simulink model "noxiebo"  (R2018b)
settings: Solver=FixedStepDiscrete  StartTime=0.0  StopTime=Inf  FixedStep=Auto  RelTol=1e-3  EnableMultiTasking=on
model workspace (MAT data in the model file):
  encoderResolution = 4096
  indexOffset = 0
  polePairs = 16
undefined symbols (not defined in the file or in its folder): Down, Up
libraries: idelinklib_common x37, c2833xlib x7, c280xlib x6, simulink x3, simulink_extras x2, c2000lib x1
(part 2 of 3)

== system noxiebo/Subsystem1/PI-Nr ==
  err : Inport
  reset : Inport  Port=2
  P : Inport  Port=3
  I : Inport  Port=4
  D : Inport  Port=5
  OV : Inport  Port=6
  Constant1 : Constant  Value=0  OutDataTypeStr=Inherit: Inherit via back propagation
  Constant2 : Constant  Value=25  OutDataTypeStr=Inherit: Inherit via back propagation
  Constant3 : Constant  Value=0  OutDataTypeStr=Inherit: Inherit via back propagation
  Constant5 : Constant  Value=0  OutDataTypeStr=Inherit: Inherit via back propagation
  Logical Operator5 : Logic  AllPortsSameDT=off  OutDataTypeStr=boolean
  Logical Operator6 : Logic  Operator=NOT  AllPortsSameDT=off  OutDataTypeStr=boolean
  Product : Product  RndMeth=Zero
  Product1 : Product  RndMeth=Zero
  Product2 : Product  RndMeth=Zero
  RC filter8 : Subsystem  mask{a=0.4}
      mask prompts: a "Time Constant"
  Saturation : Saturate  UpperLimit=max  LowerLimit=min  LinearizeAsGain=off  ZeroCross=off  OutDataTypeStr=double
  Saturation1 : Saturate  UpperLimit=ermax  LowerLimit=ermin  LinearizeAsGain=off  ZeroCross=off  OutDataTypeStr=double
  Saturation2 : Saturate  UpperLimit=max  LowerLimit=min  LinearizeAsGain=off  ZeroCross=off  OutDataTypeStr=double
  Sum1 : Sum  Inputs=+++
  Sum2 : Sum  Inputs=+-
  Sum4 : Sum
  Switch{1..4} (4 alike) : Switch  Criteria=u2 > Threshold  SaturateOnIntegerOverflow=on  InputSameDT=on
  Unit Delay1 : UnitDelay  SampleTime=-1
  Unit Delay3 : UnitDelay  SampleTime=-1
  out : Outport
  wires:
  Logical Operator6/1 -> Logical Operator5/2
  Logical Operator5/1 -> Switch4/2
  RC filter8/1(y) -> Sum1/3
  Constant3/1 -> Switch3/3
  Switch3/1 -> Switch1/3
  Saturation2/1 -> Switch3/1
  Switch1/1 -> out/1
  OV/1 -> Logical Operator6/1, Switch1/2
  Constant2/1 -> Switch1/1
  Sum1/1 -> Saturation2/1
  Product2/1 -> RC filter8/1(x)
  Unit Delay1/1 -> Sum2/2
  D/1 -> Product2/2
  Sum2/1 -> Product2/1
  Switch4/1 -> Unit Delay3/1
  Unit Delay3/1 -> Sum4/2
  Saturation/1 -> Switch4/1, Sum1/2
  Sum4/1 -> Saturation/1
  Product1/1 -> Sum4/1
  I/1 -> Product1/2
  Product/1 -> Sum1/1
  Saturation1/1 -> Switch2/1
  err/1 -> Saturation1/1
  Constant1/1 -> Switch2/3
  reset/1 -> Logical Operator5/1, Switch3/2, Switch2/2
  Switch2/1 -> Unit Delay1/1, Sum2/1, Product1/1, Product/1
  P/1 -> Product/2
  Constant5/1 -> Switch4/3

== system noxiebo/Subsystem1/RC filter1 ==
  x : Inport
  Constant2 : Constant  Value=a  OutDataTypeStr=double
  Constant3 : Constant  Value=1-a  OutDataTypeStr=double
  Divide : Product
  Divide1 : Product
  Sum2 : Sum
  Unit Delay2 : UnitDelay  SampleTime=-1
  y : Outport
  wires:
  x/1 -> Divide/1
  Constant2/1 -> Divide/2
  Constant3/1 -> Divide1/1
  Divide/1 -> Sum2/1
  Divide1/1 -> Sum2/2
  Sum2/1 -> y/1, Unit Delay2/1
  Unit Delay2/1 -> Divide1/2

== system noxiebo/Subsystem1/RC filter2 ==
  x : Inport
  Constant2 : Constant  Value=a  OutDataTypeStr=double
  Constant3 : Constant  Value=1-a  OutDataTypeStr=double
  Divide : Product
  Divide1 : Product
  Sum2 : Sum
  Unit Delay2 : UnitDelay  SampleTime=-1
  y : Outport
  wires:
  Unit Delay2/1 -> Divide1/2
  Sum2/1 -> Unit Delay2/1, y/1
  Divide1/1 -> Sum2/2
  Divide/1 -> Sum2/1
  Constant3/1 -> Divide1/1
  Constant2/1 -> Divide/2
  x/1 -> Divide/1

== system noxiebo/Subsystem1/RC filter3 ==
  x : Inport
  Constant2 : Constant  Value=a  OutDataTypeStr=double
  Constant3 : Constant  Value=1-a  OutDataTypeStr=double
  Divide : Product
  Divide1 : Product
  Sum2 : Sum
  Unit Delay2 : UnitDelay  SampleTime=-1
  y : Outport
  wires:
  Unit Delay2/1 -> Divide1/2
  Sum2/1 -> Unit Delay2/1, y/1
  Divide1/1 -> Sum2/2
  Divide/1 -> Sum2/1
  Constant3/1 -> Divide1/1
  Constant2/1 -> Divide/2
  x/1 -> Divide/1

== system noxiebo/Subsystem1/RC filter4 ==
  x : Inport
  Constant2 : Constant  Value=a  OutDataTypeStr=double
  Constant3 : Constant  Value=1-a  OutDataTypeStr=double
  Divide : Product
  Divide1 : Product
  Sum2 : Sum
  Unit Delay2 : UnitDelay  SampleTime=-1
  y : Outport
  wires:
  x/1 -> Divide/1
  Constant2/1 -> Divide/2
  Constant3/1 -> Divide1/1
  Divide/1 -> Sum2/1
  Divide1/1 -> Sum2/2
  Sum2/1 -> y/1, Unit Delay2/1
  Unit Delay2/1 -> Divide1/2

== system noxiebo/Subsystem1/RC filter5 ==
  x : Inport
  Constant2 : Constant  Value=a  OutDataTypeStr=double
  Constant3 : Constant  Value=1-a  OutDataTypeStr=double
  Divide : Product
  Divide1 : Product
  Sum2 : Sum
  Unit Delay2 : UnitDelay  SampleTime=-1
  y : Outport
  wires:
  Unit Delay2/1 -> Divide1/2
  Sum2/1 -> Unit Delay2/1, y/1
  Divide1/1 -> Sum2/2
  Divide/1 -> Sum2/1
  Constant3/1 -> Divide1/1
  Constant2/1 -> Divide/2
  x/1 -> Divide/1

== system noxiebo/Subsystem1/RC filter9 ==
  x : Inport
  Constant2 : Constant  Value=a  OutDataTypeStr=double
  Constant3 : Constant  Value=1-a  OutDataTypeStr=double
  Divide : Product
  Divide1 : Product
  Sum2 : Sum
  Unit Delay2 : UnitDelay  SampleTime=-1
  y : Outport
  wires:
  Unit Delay2/1 -> Divide1/2
  Sum2/1 -> Unit Delay2/1, y/1
  Divide1/1 -> Sum2/2
  Divide/1 -> Sum2/1
  Constant3/1 -> Divide1/1
  Constant2/1 -> Divide/2
  x/1 -> Divide/1

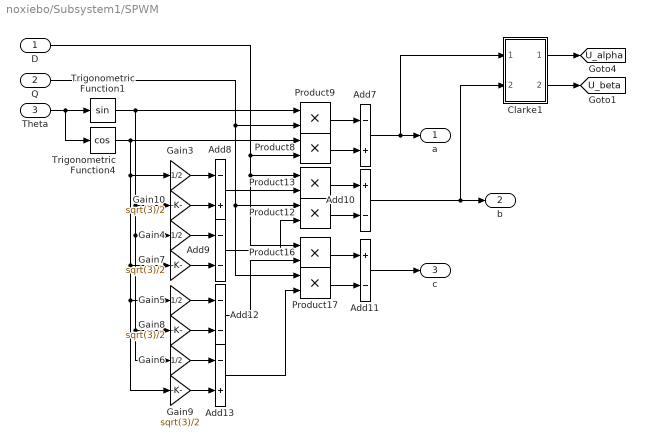
== system noxiebo/Subsystem1/SPWM ==
  D : Inport
  Q : Inport  Port=2
  Theta : Inport  Port=3
  Add10 : Sum  Inputs=+-
  Add11 : Sum  Inputs=+-
  Add12 : Sum  Inputs=--
  Add13 : Sum  Inputs=-+
  Add7 : Sum  Inputs=-+
  Add8 : Sum  Inputs=-+
  Add9 : Sum  Inputs=--
  Clarke1 : Subsystem
  Gain{7..10} (4 alike) : Gain  Gain=sqrt(3)/2
  Gain{3..6} (4 alike) : Gain  Gain=1/2
  Product{8..9,12..13,16..17} (6 alike) : Product  RndMeth=Zero
  Trigonometric Function1 : Trigonometry
  Trigonometric Function4 : Trigonometry  Operator=cos
  a : Outport
  b : Outport  Port=2
  c : Outport  Port=3
  tag scope: U_alpha=global, U_beta=global
  wires:
  Theta/1 -> Trigonometric Function1/1, Trigonometric Function4/1
  Trigonometric Function4/1 -> Product8/1, Gain3/1, Gain5/1, Gain9/1, Gain7/1
  Product8/1 -> Add7/2
  Trigonometric Function1/1 -> Product9/1, Gain4/1, Gain6/1, Gain8/1, Gain10/1
  Product9/1 -> Add7/1
  Gain3/1 -> Add8/1
  Gain4/1 -> Add9/1
  Gain7/1 -> Add9/2
  Product13/1 -> Add10/1
  Product12/1 -> Add10/2
  Add8/1 -> Product13/2
  Add9/1 -> Product12/2
  Product16/1 -> Add11/1
  Product17/1 -> Add11/2
  Add12/1 -> Product16/2
  Add13/1 -> Product17/2
  Add7/1 -> a/1, Clarke1/1(In1)
  Add10/1 -> b/1, Clarke1/2(In2)
  Add11/1 -> c/1
  Gain6/1 -> Add13/1
  Gain8/1 -> Add12/2
  Gain5/1 -> Add12/1
  Gain9/1 -> Add13/2
  Gain10/1 -> Add8/2
  D/1 -> Product8/2, Product13/1, Product16/1
  Q/1 -> Product9/2, Product12/1, Product17/1
  Clarke1/1(alpha) -> [U_alpha]
  Clarke1/2(beta) -> [U_beta]

== system noxiebo/Subsystem1/SPWM_5 ==
  D : Inport
  Q : Inport  Port=2
  Theta : Inport  Port=3
  Add10 : Sum  Inputs=+-
  Add11 : Sum  Inputs=+-
  Add12 : Sum  Inputs=--
  Add13 : Sum  Inputs=-+
  Add7 : Sum  Inputs=-+
  Add8 : Sum  Inputs=-+
  Add9 : Sum  Inputs=--
  Gain{7..10} (4 alike) : Gain  Gain=sqrt(3)/2
  Gain{3..6} (4 alike) : Gain  Gain=1/2
  Product{8..9,12..13,16..17} (6 alike) : Product  RndMeth=Zero
  Trigonometric Function1 : Trigonometry
  Trigonometric Function4 : Trigonometry  Operator=cos
  a : Outport
  b : Outport  Port=2
  c : Outport  Port=3
  wires:
  Q/1 -> Product17/1, Product12/1, Product9/2
  D/1 -> Product16/1, Product13/1, Product8/2
  Gain10/1 -> Add8/2
  Gain9/1 -> Add13/2
  Gain5/1 -> Add12/1
  Gain8/1 -> Add12/2
  Gain6/1 -> Add13/1
  Add11/1 -> c/1
  Add10/1 -> b/1
  Add7/1 -> a/1
  Add13/1 -> Product17/2
  Add12/1 -> Product16/2
  Product17/1 -> Add11/2
  Product16/1 -> Add11/1
  Add9/1 -> Product12/2
  Add8/1 -> Product13/2
  Product12/1 -> Add10/2
  Product13/1 -> Add10/1
  Gain7/1 -> Add9/2
  Gain4/1 -> Add9/1
  Gain3/1 -> Add8/1
  Product9/1 -> Add7/1
  Trigonometric Function1/1 -> Gain10/1, Gain8/1, Gain6/1, Gain4/1, Product9/1
  Product8/1 -> Add7/2
  Trigonometric Function4/1 -> Gain7/1, Gain9/1, Gain5/1, Gain3/1, Product8/1
  Theta/1 -> Trigonometric Function4/1, Trigonometric Function1/1

== system noxiebo/Subsystem1/SPWM_7 ==
  D : Inport
  Q : Inport  Port=2
  Theta : Inport  Port=3
  Add10 : Sum  Inputs=+-
  Add11 : Sum  Inputs=+-
  Add12 : Sum  Inputs=--
  Add13 : Sum  Inputs=-+
  Add7 : Sum  Inputs=-+
  Add8 : Sum  Inputs=-+
  Add9 : Sum  Inputs=--
  Gain{7..10} (4 alike) : Gain  Gain=sqrt(3)/2
  Gain{3..6} (4 alike) : Gain  Gain=1/2
  Product{8..9,12..13,16..17} (6 alike) : Product  RndMeth=Zero
  Trigonometric Function1 : Trigonometry
  Trigonometric Function4 : Trigonometry  Operator=cos
  a : Outport
  b : Outport  Port=2
  c : Outport  Port=3
  wires:
  Q/1 -> Product17/1, Product12/1, Product9/2
  D/1 -> Product16/1, Product13/1, Product8/2
  Gain10/1 -> Add8/2
  Gain9/1 -> Add13/2
  Gain5/1 -> Add12/1
  Gain8/1 -> Add12/2
  Gain6/1 -> Add13/1
  Add11/1 -> c/1
  Add10/1 -> b/1
  Add7/1 -> a/1
  Add13/1 -> Product17/2
  Add12/1 -> Product16/2
  Product17/1 -> Add11/2
  Product16/1 -> Add11/1
  Add9/1 -> Product12/2
  Add8/1 -> Product13/2
  Product12/1 -> Add10/2
  Product13/1 -> Add10/1
  Gain7/1 -> Add9/2
  Gain4/1 -> Add9/1
  Gain3/1 -> Add8/1
  Product9/1 -> Add7/1
  Trigonometric Function1/1 -> Gain10/1, Gain8/1, Gain6/1, Gain4/1, Product9/1
  Product8/1 -> Add7/2
  Trigonometric Function4/1 -> Gain7/1, Gain9/1, Gain5/1, Gain3/1, Product8/1
  Theta/1 -> Trigonometric Function4/1, Trigonometric Function1/1

== system noxiebo/Subsystem1/Subsystem2 ==
  In1 : Inport
  In2 : Inport  Port=2
  Product : Product  RndMeth=Zero
  Product1 : Product  RndMeth=Zero
  Sqrt : Sqrt  SaturateOnIntegerOverflow=on
  Sum17 : Sum
  Out1 : Outport
  wires:
  Product/1 -> Sum17/1
  Product1/1 -> Sum17/2
  Sum17/1 -> Sqrt/1
  In1/1 -> Product/2, Product/1
  In2/1 -> Product1/2, Product1/1
  Sqrt/1 -> Out1/1

== system noxiebo/Subsystem1/abc//dq current ==
  iga : Inport
  igb : Inport  Port=2
  angle : Inport  Port=3
  Clarke1 : Subsystem
  Park1 : Subsystem
  igd : Outport
  igq : Outport  Port=2
  tag scope: i_alpha=global, i_beta=global
  wires:
  Park1/1(d) -> igd/1
  iga/1 -> Clarke1/1(In1)
  Park1/2(q) -> igq/1
  igb/1 -> Clarke1/2(In2)
  Clarke1/1(alpha) -> Park1/1(alpha), [i_alpha]
  Clarke1/2(beta) -> Park1/2(beta), [i_beta]
  angle/1 -> Park1/3(theta)

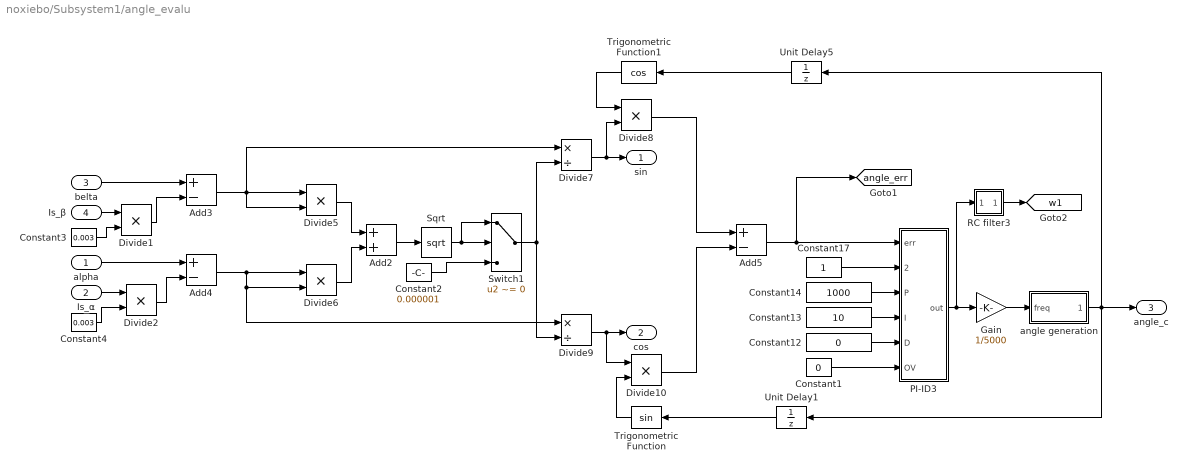
== system noxiebo/Subsystem1/angle_evalu ==
  alpha : Inport
  Is_α : Inport  Port=2
  belta : Inport  Port=3
  Is_β : Inport  Port=4
  Add2 : Sum
  Add3 : Sum  Inputs=+-
  Add4 : Sum  Inputs=+-
  Add5 : Sum  Inputs=+-
  Constant1 : Constant  Value=0  OutDataTypeStr=double
  Constant12 : Constant  Value=0  OutDataTypeStr=double
  Constant13 : Constant  Value=10  OutDataTypeStr=double
  Constant14 : Constant  Value=1000  OutDataTypeStr=double
  Constant17 : Constant  OutDataTypeStr=double
  Constant2 : Constant  Value=0.000001  OutDataTypeStr=double
  Constant3 : Constant  Value=0.003  OutDataTypeStr=double
  Constant4 : Constant  Value=0.003  OutDataTypeStr=double
  Divide{1..2,5..6,8,10} (6 alike) : Product  Inputs=**
  Divide7 : Product  Inputs=*/
  Divide9 : Product  Inputs=*/
  Gain : Gain  Gain=1/5000
  PI-ID3 : Subsystem  mask{ermax=0.5*pi, ermin=-0.5*pi, max=500, min=-500}
      mask prompts: ermax "Err max limit"; ermin "Err min limit"; max "Output max limit"; min "Output min limit"
  RC filter3 : Subsystem  mask{a=0.8}
      mask prompts: a "Time Constant"
  Sqrt : Sqrt  SaturateOnIntegerOverflow=on
  Switch1 : Switch  Criteria=u2 ~= 0
  Trigonometric Function : Trigonometry
  Trigonometric Function1 : Trigonometry  Operator=cos
  Unit Delay1 : UnitDelay  SampleTime=-1
  Unit Delay5 : UnitDelay  SampleTime=-1
  angle generation : Subsystem
  sin : Outport
  cos : Outport  Port=2
  angle_c : Outport  Port=3
  tag scope: angle_err=global, w1=global
  wires:
  belta/1 -> Add3/1
  Add3/1 -> Divide5/1, Divide5/2, Divide7/1
  Divide1/1 -> Add3/2
  Divide2/1 -> Add4/2
  Is_β/1 -> Divide1/1
  Is_α/1 -> Divide2/1
  Add4/1 -> Divide6/1, Divide6/2, Divide9/1
  Divide5/1 -> Add2/1
  Divide6/1 -> Add2/2
  Add2/1 -> Sqrt/1
  Divide7/1 -> sin/1, Divide8/2
  Divide9/1 -> cos/1, Divide10/1
  Trigonometric Function/1 -> Divide10/2
  Divide8/1 -> Add5/1
  Divide10/1 -> Add5/2
  Add5/1 -> PI-ID3/1(err), [angle_err]
  Constant17/1 -> PI-ID3/2(reset)
  Constant12/1 -> PI-ID3/5(D)
  Constant1/1 -> PI-ID3/6(OV)
  Constant14/1 -> PI-ID3/3(P)
  Constant13/1 -> PI-ID3/4(I)
  Gain/1 -> angle generation/1(freq)
  PI-ID3/1(out) -> Gain/1, RC filter3/1(x)
  angle generation/1(angle_0) -> Unit Delay5/1, Unit Delay1/1, angle_c/1
  Unit Delay5/1 -> Trigonometric Function1/1
  Unit Delay1/1 -> Trigonometric Function/1
  Trigonometric Function1/1 -> Divide8/1
  Sqrt/1 -> Switch1/2, Switch1/1
  Constant2/1 -> Switch1/3
  Switch1/1 -> Divide7/2, Divide9/2
  RC filter3/1(y) -> [w1]
  alpha/1 -> Add4/1
  Constant3/1 -> Divide1/2
  Constant4/1 -> Divide2/2

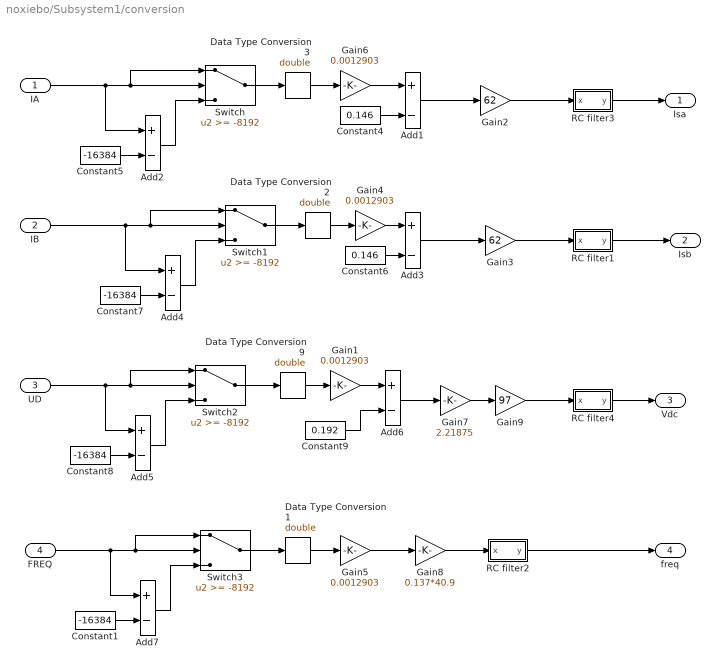
== system noxiebo/Subsystem1/conversion ==
  IA : Inport
  IB : Inport  Port=2
  UD : Inport  Port=3
  FREQ : Inport  Port=4
  Add{1..7} (7 alike) : Sum  Inputs=+-
  Constant{1,5,7..8} (4 alike) : Constant  Value=-16384  OutDataTypeStr=int16
  Constant4 : Constant  Value=0.146  OutDataTypeStr=double
  Constant6 : Constant  Value=0.146  OutDataTypeStr=double
  Constant9 : Constant  Value=0.192  OutDataTypeStr=double
  Data Type Conversion{1..3,9} (4 alike) : DataTypeConversion  OutDataTypeStr=double
  Gain{1,4..6} (4 alike) : Gain  Gain=0.0012903
  Gain2 : Gain  Gain=62
  Gain3 : Gain  Gain=62
  Gain7 : Gain  Gain=2.21875
  Gain8 : Gain  Gain=0.137*40.9
  Gain9 : Gain  Gain=97
  RC filter1 : Subsystem  mask{a=0.2}
      mask prompts: a "Time Constant"
  RC filter2 : Subsystem  mask{a=0.1}
      mask prompts: a "Time Constant"
  RC filter3 : Subsystem  mask{a=0.2}
      mask prompts: a "Time Constant"
  RC filter4 : Subsystem  mask{a=0.1}
      mask prompts: a "Time Constant"
  Switch{,1..3} (4 alike) : Switch  Threshold=-8192
  Isa : Outport
  Isb : Outport  Port=2
  Vdc : Outport  Port=3
  freq : Outport  Port=4
  wires:
  UD/1 -> Switch2/1, Switch2/2, Add5/1
  IA/1 -> Switch/1, Switch/2, Add2/1
  Constant5/1 -> Add2/2
  Add2/1 -> Switch/3
  Switch/1 -> Data Type Conversion3/1
  Data Type Conversion3/1 -> Gain6/1
  Gain2/1 -> RC filter3/1(x)
  Add1/1 -> Gain2/1
  Gain6/1 -> Add1/1
  Constant4/1 -> Add1/2
  IB/1 -> Switch1/1, Switch1/2, Add4/1
  Constant7/1 -> Add4/2
  Add4/1 -> Switch1/3
  Switch1/1 -> Data Type Conversion2/1
  Data Type Conversion2/1 -> Gain4/1
  Add3/1 -> Gain3/1
  Gain4/1 -> Add3/1
  Constant6/1 -> Add3/2
  Data Type Conversion9/1 -> Gain1/1
  Gain7/1 -> Gain9/1
  Constant8/1 -> Add5/2
  Add5/1 -> Switch2/3
  Switch2/1 -> Data Type Conversion9/1
  Gain1/1 -> Add6/1
  Add6/1 -> Gain7/1
  Constant9/1 -> Add6/2
  FREQ/1 -> Switch3/1, Switch3/2, Add7/1
  Data Type Conversion1/1 -> Gain5/1
  Constant1/1 -> Add7/2
  Add7/1 -> Switch3/3
  Switch3/1 -> Data Type Conversion1/1
  Gain5/1 -> Gain8/1
  RC filter2/1(y) -> freq/1
  Gain8/1 -> RC filter2/1(x)
  RC filter1/1(y) -> Isb/1
  RC filter3/1(y) -> Isa/1
  RC filter4/1(y) -> Vdc/1
  Gain9/1 -> RC filter4/1(x)
  Gain3/1 -> RC filter1/1(x)

== system noxiebo/Subsystem1/dq_5 ==
  alpha : Inport
  beta : Inport  Port=2
  theta : Inport  Port=3
  Add4 : Sum
  Add5 : Sum
  Gain1 : Gain  Gain=-1
  Product{,1..3} (4 alike) : Product  RndMeth=Zero
  cos : Trigonometry  Operator=cos
  sin : Trigonometry
  d : Outport
  q : Outport  Port=2
  wires:
  sin/1 -> Product2/1, Product/1
  beta/1 -> Product3/2, Product/2
  cos/1 -> Product3/1, Product1/2
  Add5/1 -> q/1
  theta/1 -> sin/1, cos/1
  Add4/1 -> d/1
  alpha/1 -> Product2/2, Product1/1
  Product1/1 -> Add4/1
  Product/1 -> Add4/2
  Product2/1 -> Gain1/1
  Gain1/1 -> Add5/1
  Product3/1 -> Add5/2

== system noxiebo/Subsystem1/dq_7 ==
  alpha : Inport
  beta : Inport  Port=2
  theta : Inport  Port=3
  Add4 : Sum
  Add5 : Sum
  Gain1 : Gain  Gain=-1
  Product{,1..3} (4 alike) : Product  RndMeth=Zero
  cos : Trigonometry  Operator=cos
  sin : Trigonometry
  d : Outport
  q : Outport  Port=2
  wires:
  sin/1 -> Product2/1, Product/1
  beta/1 -> Product3/2, Product/2
  cos/1 -> Product3/1, Product1/2
  Add5/1 -> q/1
  theta/1 -> sin/1, cos/1
  Add4/1 -> d/1
  alpha/1 -> Product2/2, Product1/1
  Product1/1 -> Add4/1
  Product/1 -> Add4/2
  Product2/1 -> Gain1/1
  Gain1/1 -> Add5/1
  Product3/1 -> Add5/2

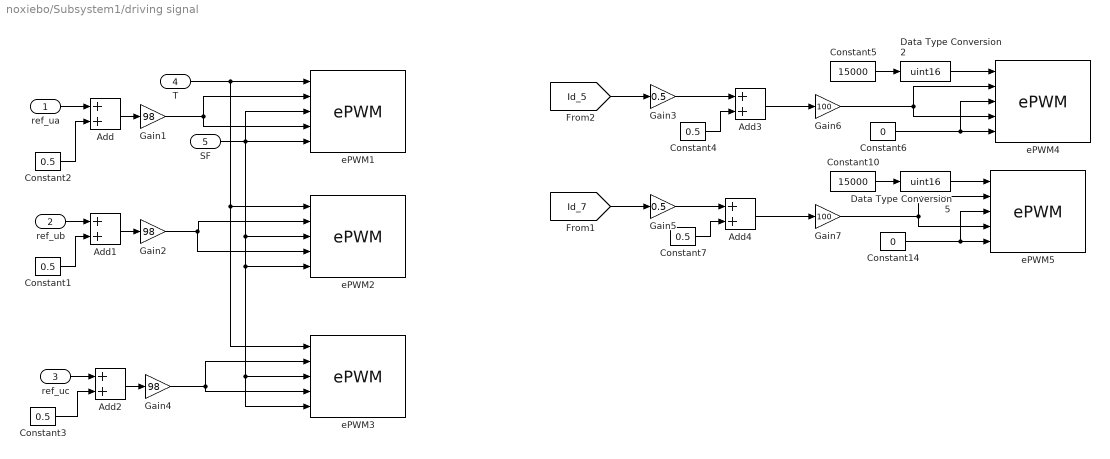
== system noxiebo/Subsystem1/driving signal ==
  ref_ua : Inport
  ref_ub : Inport  Port=2
  ref_uc : Inport  Port=3
  T : Inport  Port=4
  SF : Inport  Port=5
  Add{,1..4} (5 alike) : Sum
  Constant{1..4,7} (5 alike) : Constant  Value=0.5  OutDataTypeStr=double
  Constant10 : Constant  Value=15000  OutDataTypeStr=int16
  Constant14 : Constant  Value=0  OutDataTypeStr=boolean
  Constant5 : Constant  Value=15000  OutDataTypeStr=int16
  Constant6 : Constant  Value=0  OutDataTypeStr=boolean
  Data Type Conversion2 : DataTypeConversion  OutDataTypeStr=uint16
  Data Type Conversion5 : DataTypeConversion  OutDataTypeStr=uint16
  Gain1 : Gain  Gain=98
  Gain2 : Gain  Gain=98
  Gain3 : Gain  Gain=0.5
  Gain4 : Gain  Gain=98
  Gain5 : Gain  Gain=0.5
  Gain6 : Gain  Gain=100
  Gain7 : Gain  Gain=100
  ePWM1 : c280xlib/ePWM  checkMode=off  useModule=ePWM1  periodUnits=Clock cycles  timerSource=Input port  timerPeriod_clk=15000  timerPeriod_sec=1/20000  tbshadow=Counter equals to zero  countingMode=Up-Down  phaseActiveEnable=Disable  phaseDirection=Count down after sync  phaseActive=0  synchronizationEnable=off  synchronizationOption=Counter equals to zero (CTR=Zero)  clockPrescale=1  HSclockPrescale=1  ePWMxAStatus=off  CMPAUnits=Percentages  CMPASource=Input port  CMPAValue_per=0  CMPAValue_clk=32000  enCMPAshadow=Counter equals to zero  ePWMxAactionLogic1=Do nothing  ePWMxAactionLogic2=Do nothing  ePWMxAactionLogic3=Clear  ePWMxAactionLogic4=Set  ePWMxAactionLogic5=Do nothing  ePWMxAactionLogic6=Do nothing  ePWMxALoadMode=Load on counter equals to zero (CTR=Zero)  ePWMxACSFenable=on  ePWMxACSFvalue=Forcing disable  ePWMxASFreload=Zero  enHRPWM=off  HRPWM_LoadMode=Counter equals to zero (CTR=ZERO)  HRPWM_CTLMode=Phase control mode  HRPWM_EDGMode=Both edge  enSFO=on  ePWMxBStatus=on  CMPBUnits=Percentages  CMPBSource=Input port  CMPBValue_per=0  CMPBValue_clk=32000  enCMPBshadow=Counter equals to zero  ePWMxBactionLogic1=Do nothing  ePWMxBactionLogic2=Do nothing  ePWMxBactionLogic3=Do nothing  ePWMxBactionLogic4=Do nothing  ePWMxBactionLogic5=Set  ePWMxBactionLogic6=Clear  ePWMxBLoadMode=Load on counter equals to zero (CTR=Zero)  ePWMxBCSFenable=on  ePWMxBCSFvalue=Forcing disable  ePWMxBSFreload=Zero  enableDBePWMxA=on  enableDBePWMxB=on  DBpolarity=Active high complementary (AHC)  DBedgeDelay=Positive  DBSource_ePWMxA=ePWMxB  DBSource_ePWMxB=ePWMxB  DBperiodSource=Specify via dialog  REDperiod=525  FEDperiod=525  adcstartModuleA=off  adcrequestEventA=First event  adcstartEventA=Counter equals to zero (CTR=Zero)  adcstartModuleB=off  adcrequestEventB=First event  adcstartEventB=Counter equals to zero (CTR=Zero)  intEn=on  intPrd=First event  intSel=Counter equals to zero (CTR=Zero)  chopperEnable=off  chopperFrequency=1  chopperFirstwidth=1  chopperDuty=12.5%  tripZonesource=Specify via dialog  tzselOSHT1=off  tzselOSHT2=off  tzselOSHT3=off  tzselOSHT4=off  tzselOSHT5=off  tzselOSHT6=off  tzselCBC1=off  tzselCBC2=off  tzselCBC3=off  tzselCBC4=off  tzselCBC5=off  tzselCBC6=off  enTzOstIntr=off  enTzCbcIntr=off  ePWMxAforced=No action  ePWMxBforced=No action  timerPeriod=-1  ePWMxAValue=0  ePWMxBValue=0  tripZoneoption=One-shot trip (OSHT)
      settings: SourceProductName=Embedded Coder Support Package for Texas Instruments C2000 Processors  SourceProductBaseCode=TIC2000
  ePWM2 : c280xlib/ePWM  checkMode=off  useModule=ePWM2  periodUnits=Clock cycles  timerSource=Input port  timerPeriod_clk=15000  timerPeriod_sec=1/20000  tbshadow=Counter equals to zero  countingMode=Up-Down  phaseActiveEnable=Set counter to phase value specified via dialog  phaseDirection=Count up after sync  phaseActive=0  synchronizationEnable=off  synchronizationOption=Pass through (EPWMxSYNCI or SWFSYNC)  clockPrescale=1  HSclockPrescale=1  ePWMxAStatus=off  CMPAUnits=Percentages  CMPASource=Input port  CMPAValue_per=0  CMPAValue_clk=32000  enCMPAshadow=Counter equals to zero  ePWMxAactionLogic1=Do nothing  ePWMxAactionLogic2=Do nothing  ePWMxAactionLogic3=Clear  ePWMxAactionLogic4=Set  ePWMxAactionLogic5=Do nothing  ePWMxAactionLogic6=Do nothing  ePWMxALoadMode=Load on counter equals to zero (CTR=Zero)  ePWMxACSFenable=on  ePWMxACSFvalue=Forcing disable  ePWMxASFreload=Zero  enHRPWM=off  HRPWM_LoadMode=Counter equals to zero (CTR=ZERO)  HRPWM_CTLMode=Phase control mode  HRPWM_EDGMode=Both edge  enSFO=on  ePWMxBStatus=on  CMPBUnits=Percentages  CMPBSource=Input port  CMPBValue_per=0  CMPBValue_clk=32000  enCMPBshadow=Counter equals to zero  ePWMxBactionLogic1=Do nothing  ePWMxBactionLogic2=Do nothing  ePWMxBactionLogic3=Do nothing  ePWMxBactionLogic4=Do nothing  ePWMxBactionLogic5=Set  ePWMxBactionLogic6=Clear  ePWMxBLoadMode=Load on counter equals to zero (CTR=Zero)  ePWMxBCSFenable=on  ePWMxBCSFvalue=Forcing disable  ePWMxBSFreload=Zero  enableDBePWMxA=on  enableDBePWMxB=on  DBpolarity=Active high complementary (AHC)  DBedgeDelay=Positive  DBSource_ePWMxA=ePWMxB  DBSource_ePWMxB=ePWMxB  DBperiodSource=Specify via dialog  REDperiod=525  FEDperiod=525  adcstartModuleA=off  adcrequestEventA=First event  adcstartEventA=Counter equals to zero (CTR=Zero)  adcstartModuleB=off  adcrequestEventB=First event  adcstartEventB=Counter equals to zero (CTR=Zero)  intEn=off  intPrd=First event  intSel=Counter equals to zero (CTR=Zero)  chopperEnable=off  chopperFrequency=1  chopperFirstwidth=1  chopperDuty=12.5%  tripZonesource=Specify via dialog  tzselOSHT1=off  tzselOSHT2=off  tzselOSHT3=off  tzselOSHT4=off  tzselOSHT5=off  tzselOSHT6=off  tzselCBC1=off  tzselCBC2=off  tzselCBC3=off  tzselCBC4=off  tzselCBC5=off  tzselCBC6=off  enTzOstIntr=off  enTzCbcIntr=off  ePWMxAforced=No action  ePWMxBforced=No action  timerPeriod=-1  ePWMxAValue=0  ePWMxBValue=0  tripZoneoption=One-shot trip (OSHT)
      settings: SourceProductName=Embedded Coder Support Package for Texas Instruments C2000 Processors  SourceProductBaseCode=TIC2000
  ePWM3 : c280xlib/ePWM  checkMode=off  useModule=ePWM3  periodUnits=Clock cycles  timerSource=Input port  timerPeriod_clk=15000  timerPeriod_sec=1/20000  tbshadow=Counter equals to zero  countingMode=Up-Down  phaseActiveEnable=Set counter to phase value specified via dialog  phaseDirection=Count up after sync  phaseActive=0  synchronizationEnable=off  synchronizationOption=Pass through (EPWMxSYNCI or SWFSYNC)  clockPrescale=1  HSclockPrescale=1  ePWMxAStatus=off  CMPAUnits=Percentages  CMPASource=Input port  CMPAValue_per=0  CMPAValue_clk=32000  enCMPAshadow=Counter equals to zero  ePWMxAactionLogic1=Do nothing  ePWMxAactionLogic2=Do nothing  ePWMxAactionLogic3=Clear  ePWMxAactionLogic4=Set  ePWMxAactionLogic5=Do nothing  ePWMxAactionLogic6=Do nothing  ePWMxALoadMode=Load on counter equals to zero (CTR=Zero)  ePWMxACSFenable=on  ePWMxACSFvalue=Forcing disable  ePWMxASFreload=Zero  enHRPWM=off  HRPWM_LoadMode=Counter equals to zero (CTR=ZERO)  HRPWM_CTLMode=Phase control mode  HRPWM_EDGMode=Both edge  enSFO=on  ePWMxBStatus=on  CMPBUnits=Percentages  CMPBSource=Input port  CMPBValue_per=0  CMPBValue_clk=32000  enCMPBshadow=Counter equals to zero  ePWMxBactionLogic1=Do nothing  ePWMxBactionLogic2=Do nothing  ePWMxBactionLogic3=Do nothing  ePWMxBactionLogic4=Do nothing  ePWMxBactionLogic5=Set  ePWMxBactionLogic6=Clear  ePWMxBLoadMode=Load on counter equals to zero (CTR=Zero)  ePWMxBCSFenable=on  ePWMxBCSFvalue=Forcing disable  ePWMxBSFreload=Zero  enableDBePWMxA=on  enableDBePWMxB=on  DBpolarity=Active high complementary (AHC)  DBedgeDelay=Positive  DBSource_ePWMxA=ePWMxB  DBSource_ePWMxB=ePWMxB  DBperiodSource=Specify via dialog  REDperiod=525  FEDperiod=525  adcstartModuleA=off  adcrequestEventA=First event  adcstartEventA=Counter equals to zero (CTR=Zero)  adcstartModuleB=off  adcrequestEventB=First event  adcstartEventB=Counter equals to zero (CTR=Zero)  intEn=off  intPrd=First event  intSel=Counter equals to zero (CTR=Zero)  chopperEnable=off  chopperFrequency=1  chopperFirstwidth=1  chopperDuty=12.5%  tripZonesource=Specify via dialog  tzselOSHT1=off  tzselOSHT2=off  tzselOSHT3=off  tzselOSHT4=off  tzselOSHT5=off  tzselOSHT6=off  tzselCBC1=off  tzselCBC2=off  tzselCBC3=off  tzselCBC4=off  tzselCBC5=off  tzselCBC6=off  enTzOstIntr=off  enTzCbcIntr=off  ePWMxAforced=No action  ePWMxBforced=No action  timerPeriod=-1  ePWMxAValue=0  ePWMxBValue=0  tripZoneoption=One-shot trip (OSHT)
      settings: SourceProductName=Embedded Coder Support Package for Texas Instruments C2000 Processors  SourceProductBaseCode=TIC2000
  ePWM4 : c280xlib/ePWM  checkMode=off  useModule=ePWM4  periodUnits=Clock cycles  timerSource=Input port  timerPeriod_clk=15000  timerPeriod_sec=1/20000  tbshadow=Counter equals to zero  countingMode=Up-Down  phaseActiveEnable=Set counter to phase value specified via dialog  phaseDirection=Count up after sync  phaseActive=0  synchronizationEnable=off  synchronizationOption=Pass through (EPWMxSYNCI or SWFSYNC)  clockPrescale=1  HSclockPrescale=1  ePWMxAStatus=on  CMPAUnits=Percentages  CMPASource=Input port  CMPAValue_per=0  CMPAValue_clk=32000  enCMPAshadow=Counter equals to zero  ePWMxAactionLogic1=Do nothing  ePWMxAactionLogic2=Do nothing  ePWMxAactionLogic3=Clear  ePWMxAactionLogic4=Set  ePWMxAactionLogic5=Do nothing  ePWMxAactionLogic6=Do nothing  ePWMxALoadMode=Load on counter equals to zero (CTR=Zero)  ePWMxACSFenable=on  ePWMxACSFvalue=Forcing disable  ePWMxASFreload=Zero  enHRPWM=off  HRPWM_LoadMode=Counter equals to zero (CTR=ZERO)  HRPWM_CTLMode=Phase control mode  HRPWM_EDGMode=Both edge  enSFO=on  ePWMxBStatus=on  CMPBUnits=Percentages  CMPBSource=Input port  CMPBValue_per=0  CMPBValue_clk=32000  enCMPBshadow=Counter equals to zero  ePWMxBactionLogic1=Do nothing  ePWMxBactionLogic2=Do nothing  ePWMxBactionLogic3=Do nothing  ePWMxBactionLogic4=Do nothing  ePWMxBactionLogic5=Clear  ePWMxBactionLogic6=Set  ePWMxBLoadMode=Load on counter equals to zero (CTR=Zero)  ePWMxBCSFenable=on  ePWMxBCSFvalue=Forcing disable  ePWMxBSFreload=Zero  enableDBePWMxA=off  enableDBePWMxB=off  DBpolarity=Active high complementary (AHC)  DBedgeDelay=Positive  DBSource_ePWMxA=ePWMxB  DBSource_ePWMxB=ePWMxB  DBperiodSource=Specify via dialog  REDperiod=0  FEDperiod=0  adcstartModuleA=off  adcrequestEventA=First event  adcstartEventA=Counter equals to zero (CTR=Zero)  adcstartModuleB=off  adcrequestEventB=First event  adcstartEventB=Counter equals to zero (CTR=Zero)  intEn=off  intPrd=First event  intSel=Counter equals to zero (CTR=Zero)  chopperEnable=off  chopperFrequency=1  chopperFirstwidth=1  chopperDuty=12.5%  tripZonesource=Specify via dialog  tzselOSHT1=off  tzselOSHT2=off  tzselOSHT3=off  tzselOSHT4=off  tzselOSHT5=off  tzselOSHT6=off  tzselCBC1=off  tzselCBC2=off  tzselCBC3=off  tzselCBC4=off  tzselCBC5=off  tzselCBC6=off  enTzOstIntr=off  enTzCbcIntr=off  ePWMxAforced=No action  ePWMxBforced=No action  timerPeriod=-1  ePWMxAValue=0  ePWMxBValue=0  tripZoneoption=One-shot trip (OSHT)
      settings: SourceProductName=Embedded Coder Support Package for Texas Instruments C2000 Processors  SourceProductBaseCode=TIC2000
  ePWM5 : c280xlib/ePWM  checkMode=off  useModule=ePWM5  periodUnits=Clock cycles  timerSource=Input port  timerPeriod_clk=15000  timerPeriod_sec=1/20000  tbshadow=Counter equals to zero  countingMode=Up-Down  phaseActiveEnable=Set counter to phase value specified via dialog  phaseDirection=Count up after sync  phaseActive=0  synchronizationEnable=off  synchronizationOption=Pass through (EPWMxSYNCI or SWFSYNC)  clockPrescale=1  HSclockPrescale=1  ePWMxAStatus=on  CMPAUnits=Percentages  CMPASource=Input port  CMPAValue_per=0  CMPAValue_clk=32000  enCMPAshadow=Counter equals to zero  ePWMxAactionLogic1=Do nothing  ePWMxAactionLogic2=Do nothing  ePWMxAactionLogic3=Clear  ePWMxAactionLogic4=Set  ePWMxAactionLogic5=Do nothing  ePWMxAactionLogic6=Do nothing  ePWMxALoadMode=Load on counter equals to zero (CTR=Zero)  ePWMxACSFenable=on  ePWMxACSFvalue=Forcing disable  ePWMxASFreload=Zero  enHRPWM=off  HRPWM_LoadMode=Counter equals to zero (CTR=ZERO)  HRPWM_CTLMode=Phase control mode  HRPWM_EDGMode=Both edge  enSFO=on  ePWMxBStatus=on  CMPBUnits=Percentages  CMPBSource=Input port  CMPBValue_per=0  CMPBValue_clk=32000  enCMPBshadow=Counter equals to zero  ePWMxBactionLogic1=Do nothing  ePWMxBactionLogic2=Do nothing  ePWMxBactionLogic3=Do nothing  ePWMxBactionLogic4=Do nothing  ePWMxBactionLogic5=Clear  ePWMxBactionLogic6=Set  ePWMxBLoadMode=Load on counter equals to zero (CTR=Zero)  ePWMxBCSFenable=on  ePWMxBCSFvalue=Forcing disable  ePWMxBSFreload=Zero  enableDBePWMxA=off  enableDBePWMxB=off  DBpolarity=Active high complementary (AHC)  DBedgeDelay=Positive  DBSource_ePWMxA=ePWMxB  DBSource_ePWMxB=ePWMxB  DBperiodSource=Specify via dialog  REDperiod=0  FEDperiod=0  adcstartModuleA=off  adcrequestEventA=First event  adcstartEventA=Counter equals to zero (CTR=Zero)  adcstartModuleB=off  adcrequestEventB=First event  adcstartEventB=Counter equals to zero (CTR=Zero)  intEn=off  intPrd=First event  intSel=Counter equals to zero (CTR=Zero)  chopperEnable=off  chopperFrequency=1  chopperFirstwidth=1  chopperDuty=12.5%  tripZonesource=Specify via dialog  tzselOSHT1=off  tzselOSHT2=off  tzselOSHT3=off  tzselOSHT4=off  tzselOSHT5=off  tzselOSHT6=off  tzselCBC1=off  tzselCBC2=off  tzselCBC3=off  tzselCBC4=off  tzselCBC5=off  tzselCBC6=off  enTzOstIntr=off  enTzCbcIntr=off  ePWMxAforced=No action  ePWMxBforced=No action  timerPeriod=-1  ePWMxAValue=0  ePWMxBValue=0  tripZoneoption=One-shot trip (OSHT)
      settings: SourceProductName=Embedded Coder Support Package for Texas Instruments C2000 Processors  SourceProductBaseCode=TIC2000
  wires:
  SF/1 -> ePWM1/3, ePWM1/5, ePWM3/5, ePWM3/3, ePWM2/5, ePWM2/3
  T/1 -> ePWM1/1, ePWM3/1, ePWM2/1
  ref_ua/1 -> Add/1
  Add/1 -> Gain1/1
  Constant2/1 -> Add/2
  Gain1/1 -> ePWM1/2, ePWM1/4
  ref_ub/1 -> Add1/1
  Constant1/1 -> Add1/2
  Add1/1 -> Gain2/1
  Gain2/1 -> ePWM2/4, ePWM2/2
  ref_uc/1 -> Add2/1
  Constant3/1 -> Add2/2
  Add2/1 -> Gain4/1
  Gain4/1 -> ePWM3/2, ePWM3/4
  Data Type Conversion5/1 -> ePWM5/1
  Constant14/1 -> ePWM5/3, ePWM5/5
  Constant5/1 -> Data Type Conversion2/1
  Gain7/1 -> ePWM5/2, ePWM5/4
  Data Type Conversion2/1 -> ePWM4/1
  Gain6/1 -> ePWM4/4, ePWM4/2
  Constant10/1 -> Data Type Conversion5/1
  Constant6/1 -> ePWM4/3, ePWM4/5
  [Id_5] -> Gain3/1
  [Id_7] -> Gain5/1
  Constant4/1 -> Add3/2
  Gain3/1 -> Add3/1
  Add3/1 -> Gain6/1
  Constant7/1 -> Add4/2
  Gain5/1 -> Add4/1
  Add4/1 -> Gain7/1

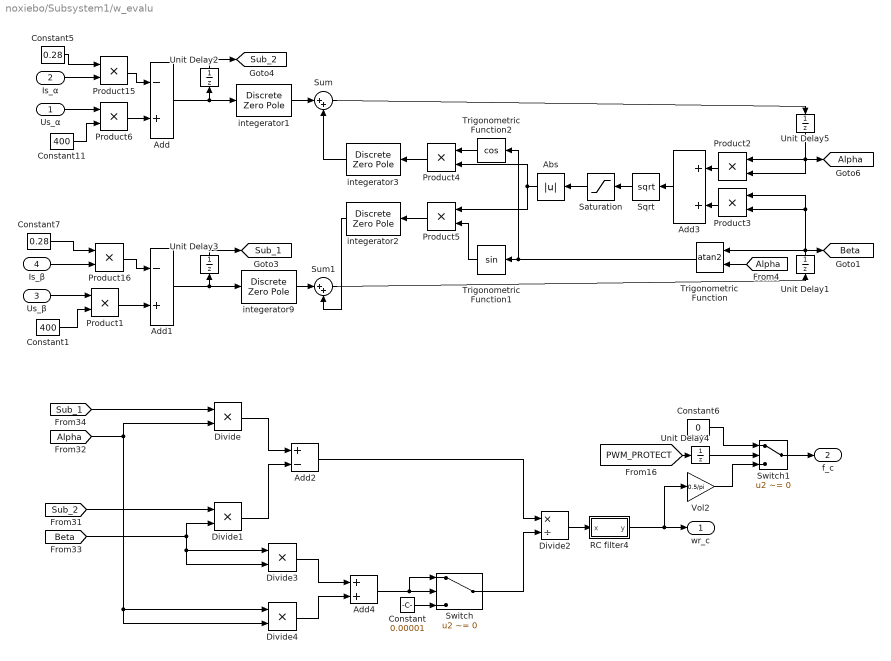
== system noxiebo/Subsystem1/w_evalu ==
  Us_α : Inport
  Is_α : Inport  Port=2
  Us_β : Inport  Port=3
  Is_β : Inport  Port=4
  Abs : Abs
  Add : Sum  Inputs=-+
  Add1 : Sum  Inputs=-+
  Add2 : Sum  Inputs=+-
  Add3 : Sum
  Add4 : Sum
  Constant : Constant  Value=0.00001
  Constant1 : Constant  Value=400  OutDataTypeStr=double
  Constant11 : Constant  Value=400  OutDataTypeStr=double
  Constant5 : Constant  Value=0.28  OutDataTypeStr=double
  Constant6 : Constant  Value=0  OutDataTypeStr=double
  Constant7 : Constant  Value=0.28  OutDataTypeStr=double
  Divide{,1,3..4} (4 alike) : Product  Inputs=**
  Divide2 : Product  Inputs=*/
  Product{1..6,15..16} (8 alike) : Product  RndMeth=Zero
  RC filter4 : Subsystem  mask{a=0.05}
      mask prompts: a "Time Constant"
  Saturation : Saturate  UpperLimit=0.56  LowerLimit=-0.56
  Sqrt : Sqrt  SaturateOnIntegerOverflow=on
  Sum : Sum  Inputs=|++
  Sum1 : Sum  Inputs=|++
  Switch : Switch  Criteria=u2 ~= 0
  Switch1 : Switch  Criteria=u2 ~= 0
  Trigonometric Function : Trigonometry  Operator=atan2
  Trigonometric Function1 : Trigonometry
  Trigonometric Function2 : Trigonometry  Operator=cos
  Unit Delay{1..5} (5 alike) : UnitDelay  SampleTime=-1
  Vol2 : Gain  Gain=0.5/pi
  integerator1 : DiscreteZeroPole  Zeros=[0]  Poles=[1/1.03]  Gain=0.0002/1.03  SampleTime=-1
  integerator2 : DiscreteZeroPole  Zeros=[0]  Poles=[1/1.03]  Gain=0.0002/1.03*150  SampleTime=-1
  integerator3 : DiscreteZeroPole  Zeros=[0]  Poles=[1/1.03]  Gain=0.0002/1.03*150  SampleTime=-1
  integerator9 : DiscreteZeroPole  Zeros=[0]  Poles=[1/1.03]  Gain=0.0002/1.03  SampleTime=-1
  wr_c : Outport
  f_c : Outport  Port=2
  tag scope: Alpha=global, Beta=global, Sub_1=global, Sub_2=global
  wires:
  Product6/1 -> Add/2
  Add/1 -> Unit Delay2/1, integerator1/1
  Us_α/1 -> Product6/1
  Is_α/1 -> Product15/2
  Product15/1 -> Add/1
  Product16/1 -> Add1/1
  Is_β/1 -> Product16/2
  Us_β/1 -> Product1/1
  Add1/1 -> integerator9/1, Unit Delay3/1
  Product1/1 -> Add1/2
  integerator1/1 -> Sum/1
  integerator9/1 -> Sum1/1
  Sum/1 -> Unit Delay5/1
  Sum1/1 -> Unit Delay1/1
  Product3/1 -> Add3/2
  Product2/1 -> Add3/1
  Add3/1 -> Sqrt/1
  Product4/1 -> integerator3/1
  Product5/1 -> integerator2/1
  Abs/1 -> Product4/2, Product5/1
  Unit Delay1/1 -> [Beta], Product3/1, Product3/2, Trigonometric Function/1
  Unit Delay5/1 -> Product2/2, Product2/1, [Alpha]
  Unit Delay2/1 -> [Sub_2]
  Unit Delay3/1 -> [Sub_1]
  Sqrt/1 -> Saturation/1
  Saturation/1 -> Abs/1
  [Alpha] -> Trigonometric Function/2
  Trigonometric Function/1 -> Trigonometric Function1/1, Trigonometric Function2/1
  Trigonometric Function1/1 -> Product5/2
  Trigonometric Function2/1 -> Product4/1
  integerator2/1 -> Sum1/2
  integerator3/1 -> Sum/2
  [Sub_1] -> Divide/1
  [Alpha] -> Divide/2, Divide4/1, Divide4/2
  [Sub_2] -> Divide1/1
  [Beta] -> Divide1/2, Divide3/1, Divide3/2
  Divide/1 -> Add2/1
  Divide1/1 -> Add2/2
  Add2/1 -> Divide2/1
  Divide3/1 -> Add4/1
  Divide4/1 -> Add4/2
  Divide2/1 -> RC filter4/1(x)
  Add4/1 -> Switch/2, Switch/1
  Switch/1 -> Divide2/2
  Constant/1 -> Switch/3
  RC filter4/1(y) -> wr_c/1, Vol2/1
  Switch1/1 -> f_c/1
  [PWM_PROTECT] -> Unit Delay4/1
  Constant6/1 -> Switch1/1
  Unit Delay4/1 -> Switch1/2
  Vol2/1 -> Switch1/3
  Constant1/1 -> Product1/2
  Constant11/1 -> Product6/2
  Constant5/1 -> Product15/1
  Constant7/1 -> Product16/1

== system noxiebo/Function-Call Subsystem1/Subsystem1/求个位 ==
  In1 : Inport
  In2 : Inport  Port=2
  In3 : Inport  Port=3
  Constant1 : Constant  OutDataTypeStr=uint16
  Gain : Gain  Gain=100
  Gain1 : Gain  Gain=10
  Math Function : Math  Operator=rem  SaturateOnIntegerOverflow=on
  Product : Product  Inputs=*/
  Sum : Sum  Inputs=+--  AccumDataTypeStr=uint16  OutDataTypeStr=uint16
  Sum1 : Sum  Inputs=+-
  Out1 : Outport
  wires:
  In2/1 -> Gain/1
  In3/1 -> Gain1/1
  In1/1 -> Sum/1
  Gain/1 -> Sum/2
  Gain1/1 -> Sum/3
  Sum1/1 -> Product/1
  Math Function/1 -> Sum1/2
  Constant1/1 -> Math Function/2, Product/2
  Product/1 -> Out1/1
  Sum/1 -> Math Function/1, Sum1/1

== system noxiebo/Function-Call Subsystem1/Subsystem1/求十位 ==
  In1 : Inport
  In2 : Inport  Port=2
  Constant1 : Constant  Value=10  OutDataTypeStr=uint16
  Gain1 : Gain  Gain=100
  Math Function : Math  Operator=rem  SaturateOnIntegerOverflow=on
  Product : Product  Inputs=*/
  Sum : Sum  Inputs=+-
  Sum1 : Sum  Inputs=+-  OutDataTypeStr=uint16
  Out1 : Outport
  wires:
  Sum/1 -> Product/1
  Math Function/1 -> Sum/2
  Constant1/1 -> Math Function/2, Product/2
  Product/1 -> Out1/1
  In1/1 -> Gain1/1
  In2/1 -> Sum1/1
  Gain1/1 -> Sum1/2
  Sum1/1 -> Sum/1, Math Function/1

== system noxiebo/Function-Call Subsystem1/Subsystem1/求百位 ==
  In1 : Inport
  Constant1 : Constant  Value=100  OutDataTypeStr=uint16
  Math Function : Math  Operator=rem  SaturateOnIntegerOverflow=on
  Product : Product  Inputs=*/
  Sum : Sum  Inputs=+-
  Out1 : Outport
  wires:
  Product/1 -> Out1/1
  Constant1/1 -> Product/2, Math Function/2
  In1/1 -> Sum/1, Math Function/1
  Math Function/1 -> Sum/2
  Sum/1 -> Product/1

== system noxiebo/Function-Call Subsystem1/Subsystem2/求个位 ==
  In1 : Inport
  In2 : Inport  Port=2
  In3 : Inport  Port=3
  Constant1 : Constant  OutDataTypeStr=uint16
  Gain : Gain  Gain=100
  Gain1 : Gain  Gain=10
  Math Function : Math  Operator=rem  SaturateOnIntegerOverflow=on
  Product : Product  Inputs=*/
  Sum : Sum  Inputs=+--  AccumDataTypeStr=uint16  OutDataTypeStr=uint16
  Sum1 : Sum  Inputs=+-
  Out1 : Outport
  wires:
  Sum/1 -> Sum1/1, Math Function/1
  Product/1 -> Out1/1
  Constant1/1 -> Product/2, Math Function/2
  Math Function/1 -> Sum1/2
  Sum1/1 -> Product/1
  Gain1/1 -> Sum/3
  Gain/1 -> Sum/2
  In1/1 -> Sum/1
  In3/1 -> Gain1/1
  In2/1 -> Gain/1

== system noxiebo/Function-Call Subsystem1/Subsystem2/求十位 ==
  In1 : Inport
  In2 : Inport  Port=2
  Constant1 : Constant  Value=10  OutDataTypeStr=uint16
  Gain1 : Gain  Gain=100
  Math Function : Math  Operator=rem  SaturateOnIntegerOverflow=on
  Product : Product  Inputs=*/
  Sum : Sum  Inputs=+-
  Sum1 : Sum  Inputs=+-  OutDataTypeStr=uint16
  Out1 : Outport
  wires:
  Sum1/1 -> Math Function/1, Sum/1
  Gain1/1 -> Sum1/2
  In2/1 -> Sum1/1
  In1/1 -> Gain1/1
  Product/1 -> Out1/1
  Constant1/1 -> Product/2, Math Function/2
  Math Function/1 -> Sum/2
  Sum/1 -> Product/1

== system noxiebo/Function-Call Subsystem1/Subsystem2/求百位 ==
  In1 : Inport
  Constant1 : Constant  Value=100  OutDataTypeStr=uint16
  Math Function : Math  Operator=rem  SaturateOnIntegerOverflow=on
  Product : Product  Inputs=*/
  Sum : Sum  Inputs=+-
  Out1 : Outport
  wires:
  Sum/1 -> Product/1
  Math Function/1 -> Sum/2
  In1/1 -> Math Function/1, Sum/1
  Constant1/1 -> Math Function/2, Product/2
  Product/1 -> Out1/1

== system noxiebo/Function-Call Subsystem1/Subsystem3/求个位 ==
  In1 : Inport
  In2 : Inport  Port=2
  In3 : Inport  Port=3
  Constant1 : Constant  OutDataTypeStr=uint16
  Gain : Gain  Gain=100
  Gain1 : Gain  Gain=10
  Math Function : Math  Operator=rem  SaturateOnIntegerOverflow=on
  Product : Product  Inputs=*/
  Sum : Sum  Inputs=+--  AccumDataTypeStr=uint16  OutDataTypeStr=uint16
  Sum1 : Sum  Inputs=+-
  Out1 : Outport
  wires:
  In2/1 -> Gain/1
  In3/1 -> Gain1/1
  In1/1 -> Sum/1
  Gain/1 -> Sum/2
  Gain1/1 -> Sum/3
  Sum1/1 -> Product/1
  Math Function/1 -> Sum1/2
  Constant1/1 -> Math Function/2, Product/2
  Product/1 -> Out1/1
  Sum/1 -> Math Function/1, Sum1/1

== system noxiebo/Function-Call Subsystem1/Subsystem3/求十位 ==
  In1 : Inport
  In2 : Inport  Port=2
  Constant1 : Constant  Value=10  OutDataTypeStr=uint16
  Gain1 : Gain  Gain=100
  Math Function : Math  Operator=rem  SaturateOnIntegerOverflow=on
  Product : Product  Inputs=*/
  Sum : Sum  Inputs=+-
  Sum1 : Sum  Inputs=+-  OutDataTypeStr=uint16
  Out1 : Outport
  wires:
  Sum/1 -> Product/1
  Math Function/1 -> Sum/2
  Constant1/1 -> Math Function/2, Product/2
  Product/1 -> Out1/1
  In1/1 -> Gain1/1
  In2/1 -> Sum1/1
  Gain1/1 -> Sum1/2
  Sum1/1 -> Sum/1, Math Function/1

== system noxiebo/Function-Call Subsystem1/Subsystem3/求百位 ==
  In1 : Inport
  Constant1 : Constant  Value=100  OutDataTypeStr=uint16
  Math Function : Math  Operator=rem  SaturateOnIntegerOverflow=on
  Product : Product  Inputs=*/
  Sum : Sum  Inputs=+-
  Out1 : Outport
  wires:
  Product/1 -> Out1/1
  Constant1/1 -> Product/2, Math Function/2
  In1/1 -> Sum/1, Math Function/1
  Math Function/1 -> Sum/2
  Sum/1 -> Product/1

== system noxiebo/Subsystem1/AD/Start Conversion ==
  Constant : Constant  Value=0  OutDataTypeStr=boolean
  Digital Output1 : c2833xlib/Digital Output  Priority=1  GPIO_Number=GPIO48~GPIO55  GPIO_Bit0=off  GPIO_BIT0_Toggle=off  GPIO_Bit1=on  GPIO_BIT1_Toggle=off  GPIO_Bit2=off  GPIO_BIT2_Toggle=off  GPIO_Bit3=off  GPIO_BIT3_Toggle=off  GPIO_Bit4=off  GPIO_BIT4_Toggle=off  GPIO_Bit5=off  GPIO_BIT5_Toggle=off  GPIO_Bit6=off  GPIO_BIT6_Toggle=off  GPIO_Bit7=off  GPIO_BIT7_Toggle=off
      settings: SourceProductName=Embedded Coder Support Package for Texas Instruments C2000 Processors  SourceProductBaseCode=TIC2000
  wires:
  Constant/1 -> Digital Output1/1

== system noxiebo/Subsystem1/AD/Stop Conversion ==
  Constant12 : Constant  OutDataTypeStr=boolean
  Digital Output13 : c2833xlib/Digital Output  Priority=8  GPIO_Number=GPIO48~GPIO55  GPIO_Bit0=off  GPIO_BIT0_Toggle=off  GPIO_Bit1=on  GPIO_BIT1_Toggle=off  GPIO_Bit2=off  GPIO_BIT2_Toggle=off  GPIO_Bit3=off  GPIO_BIT3_Toggle=off  GPIO_Bit4=off  GPIO_BIT4_Toggle=off  GPIO_Bit5=off  GPIO_BIT5_Toggle=off  GPIO_Bit6=off  GPIO_BIT6_Toggle=off  GPIO_Bit7=off  GPIO_BIT7_Toggle=off
      settings: SourceProductName=Embedded Coder Support Package for Texas Instruments C2000 Processors  SourceProductBaseCode=TIC2000
  wires:
  Constant12/1 -> Digital Output13/1
